simulink model "My_Model"  (R2022a)
settings: Solver=VariableStepAuto  StartTime=0.0  StopTime=10.0  RelTol=1e-3
libraries: neural x1294, spsSeriesRLCBranchLib x16, spsDiodeLib x14, spsMosfetLib x9, spsVoltageMeasurementLib x9, powerlib_extras x8, spsThreePhaseVIMeasurementLib x7, spsCurrentMeasurementLib x4, spsPVArrayLib x4, spsPWMGeneratorDCDCLib x4, spsTHDLib x4, spsThreePhaseParallelRLCBranchLib x3
(part 39 of 41)

== system My_Model/VSC Control/Current Regulator/7 layer network/Layer 5/IW{5,1} ==
  "pd{5,1}" : Inport  PortDimensions=2
      mask Display: e = 0.06;c1 = [120 230 180]/255;c2 = ([120 230 180]+0)/(256+128);c3 = ([120 230 180]+128)/(256+128);patch([0 1 1 0],[0 0 1 1],c1);patch([0 1 1 1-e 1-e 0+e],[0 0 1 1-e 0+e 0+e],c2);patch([0 0 1 1-e 0+e 0+e],[0 1 1 1-e 1-e 0+e],c3);plot([0 1 1 0 0],[0 0 1 1 0]);
  "IW{5,1}(1,:)'" : Constant  Value=[0.2265183678603188421885050729542854242026805877685546875;-0.080454707579343642809277525884681381285190582275390625]
      mask Display: e = 0.06;c1 = [120 150 230]/255;c2 = ([120 150 230]+0)/383;c3 = ([120 150 230]+128)/383;patch([0 1 1 0],[0 0 1 1],c1);patch([0 1 1 1-e 1-e 0+e],[0 0 1 1-e 0+e 0+e],c2);patch([0 0 1 1-e 0+e 0+e],[0 1 1 1-e 1-e 0+e],c3);plot([0 1 1 0 0],[0 0 1 1 0]);disp('Weights');
  "IW{5,1}(10,:)'" : Constant  Value=[-0.1422788353639719283183495690536801703274250030517578125;-0.07623245493874390710242749946701223962008953094482421875]
      mask Display: e = 0.06;c1 = [120 150 230]/255;c2 = ([120 150 230]+0)/383;c3 = ([120 150 230]+128)/383;patch([0 1 1 0],[0 0 1 1],c1);patch([0 1 1 1-e 1-e 0+e],[0 0 1 1-e 0+e 0+e],c2);patch([0 0 1 1-e 0+e 0+e],[0 1 1 1-e 1-e 0+e],c3);plot([0 1 1 0 0],[0 0 1 1 0]);disp('Weights');
  "IW{5,1}(2,:)'" : Constant  Value=[-0.4991813426266704656342199086793698370456695556640625;0.0282721598553938892328663001762834028340876102447509765625]
      mask Display: e = 0.06;c1 = [120 150 230]/255;c2 = ([120 150 230]+0)/383;c3 = ([120 150 230]+128)/383;patch([0 1 1 0],[0 0 1 1],c1);patch([0 1 1 1-e 1-e 0+e],[0 0 1 1-e 0+e 0+e],c2);patch([0 0 1 1-e 0+e 0+e],[0 1 1 1-e 1-e 0+e],c3);plot([0 1 1 0 0],[0 0 1 1 0]);disp('Weights');
  "IW{5,1}(3,:)'" : Constant  Value=[0.1044406469762407529966452557346201501786708831787109375;0.046202458042315097674901380742085166275501251220703125]
      mask Display: e = 0.06;c1 = [120 150 230]/255;c2 = ([120 150 230]+0)/383;c3 = ([120 150 230]+128)/383;patch([0 1 1 0],[0 0 1 1],c1);patch([0 1 1 1-e 1-e 0+e],[0 0 1 1-e 0+e 0+e],c2);patch([0 0 1 1-e 0+e 0+e],[0 1 1 1-e 1-e 0+e],c3);plot([0 1 1 0 0],[0 0 1 1 0]);disp('Weights');
  "IW{5,1}(4,:)'" : Constant  Value=[0.072802141329844138883942150641814805567264556884765625;-0.1804228821812341732044870923346024937927722930908203125]
      mask Display: e = 0.06;c1 = [120 150 230]/255;c2 = ([120 150 230]+0)/383;c3 = ([120 150 230]+128)/383;patch([0 1 1 0],[0 0 1 1],c1);patch([0 1 1 1-e 1-e 0+e],[0 0 1 1-e 0+e 0+e],c2);patch([0 0 1 1-e 0+e 0+e],[0 1 1 1-e 1-e 0+e],c3);plot([0 1 1 0 0],[0 0 1 1 0]);disp('Weights');
  "IW{5,1}(5,:)'" : Constant  Value=[-0.098564433750983615478702404288924299180507659912109375;-0.088427141857044144757082904106937348842620849609375]
      mask Display: e = 0.06;c1 = [120 150 230]/255;c2 = ([120 150 230]+0)/383;c3 = ([120 150 230]+128)/383;patch([0 1 1 0],[0 0 1 1],c1);patch([0 1 1 1-e 1-e 0+e],[0 0 1 1-e 0+e 0+e],c2);patch([0 0 1 1-e 0+e 0+e],[0 1 1 1-e 1-e 0+e],c3);plot([0 1 1 0 0],[0 0 1 1 0]);disp('Weights');
  "IW{5,1}(6,:)'" : Constant  Value=[-0.3674258864948158898044994202791713178157806396484375;0.0169846715856297354740878091661215876229107379913330078125]
      mask Display: e = 0.06;c1 = [120 150 230]/255;c2 = ([120 150 230]+0)/383;c3 = ([120 150 230]+128)/383;patch([0 1 1 0],[0 0 1 1],c1);patch([0 1 1 1-e 1-e 0+e],[0 0 1 1-e 0+e 0+e],c2);patch([0 0 1 1-e 0+e 0+e],[0 1 1 1-e 1-e 0+e],c3);plot([0 1 1 0 0],[0 0 1 1 0]);disp('Weights');
  "IW{5,1}(7,:)'" : Constant  Value=[0.4141842211099089343662171813775785267353057861328125;0.11901346031348351839351806802369537763297557830810546875]
      mask Display: e = 0.06;c1 = [120 150 230]/255;c2 = ([120 150 230]+0)/383;c3 = ([120 150 230]+128)/383;patch([0 1 1 0],[0 0 1 1],c1);patch([0 1 1 1-e 1-e 0+e],[0 0 1 1-e 0+e 0+e],c2);patch([0 0 1 1-e 0+e 0+e],[0 1 1 1-e 1-e 0+e],c3);plot([0 1 1 0 0],[0 0 1 1 0]);disp('Weights');
  "IW{5,1}(8,:)'" : Constant  Value=[-0.1725725080176267189902006293777958489954471588134765625;0.272154231131515211838944878763868473470211029052734375]
      mask Display: e = 0.06;c1 = [120 150 230]/255;c2 = ([120 150 230]+0)/383;c3 = ([120 150 230]+128)/383;patch([0 1 1 0],[0 0 1 1],c1);patch([0 1 1 1-e 1-e 0+e],[0 0 1 1-e 0+e 0+e],c2);patch([0 0 1 1-e 0+e 0+e],[0 1 1 1-e 1-e 0+e],c3);plot([0 1 1 0 0],[0 0 1 1 0]);disp('Weights');
  "IW{5,1}(9,:)'" : Constant  Value=[-0.2126507656600488405107540756944217719137668609619140625;0.11513492898073794667990199513951665721833705902099609375]
      mask Display: e = 0.06;c1 = [120 150 230]/255;c2 = ([120 150 230]+0)/383;c3 = ([120 150 230]+128)/383;patch([0 1 1 0],[0 0 1 1],c1);patch([0 1 1 1-e 1-e 0+e],[0 0 1 1-e 0+e 0+e],c2);patch([0 0 1 1-e 0+e 0+e],[0 1 1 1-e 1-e 0+e],c3);plot([0 1 1 0 0],[0 0 1 1 0]);disp('Weights');
  Mux : Mux  Inputs=10
      mask Display: e = 0.06;c1 = [120 150 230]/255;c2 = ([120 150 230]+0)/383;c3 = ([120 150 230]+128)/383;patch([0 1 1 0],[0 0 1 1],c1);patch([0 1 1 1-e 1-e 0+e],[0 0 1 1-e 0+e 0+e],c2);patch([0 0 1 1-e 0+e 0+e],[0 1 1 1-e 1-e 0+e],c3);plot([0 1 1 0 0],[0 0 1 1 0]);disp('Mux');
  dotprod{1..10} (10 alike) : neural/Weight Functions/dotprod
  "iz{5,1}" : Outport
      mask Display: e = 0.06;c1 = [120 230 180]/255;c2 = ([120 230 180]+0)/(256+128);c3 = ([120 230 180]+128)/(256+128);patch([0 1 1 0],[0 0 1 1],c1);patch([0 1 1 1-e 1-e 0+e],[0 0 1 1-e 0+e 0+e],c2);patch([0 0 1 1-e 0+e 0+e],[0 1 1 1-e 1-e 0+e],c3);plot([0 1 1 0 0],[0 0 1 1 0]);
  wires:
  "IW{5,1}(1,:)'"/1 -> dotprod1/1
  "pd{5,1}"/1 -> dotprod1/2, dotprod2/2, dotprod3/2, dotprod4/2, dotprod5/2, dotprod6/2, dotprod7/2, dotprod8/2, dotprod9/2, dotprod10/2
  dotprod1/1 -> Mux/1
  "IW{5,1}(2,:)'"/1 -> dotprod2/1
  dotprod2/1 -> Mux/2
  "IW{5,1}(3,:)'"/1 -> dotprod3/1
  dotprod3/1 -> Mux/3
  "IW{5,1}(4,:)'"/1 -> dotprod4/1
  dotprod4/1 -> Mux/4
  "IW{5,1}(5,:)'"/1 -> dotprod5/1
  dotprod5/1 -> Mux/5
  "IW{5,1}(6,:)'"/1 -> dotprod6/1
  dotprod6/1 -> Mux/6
  "IW{5,1}(7,:)'"/1 -> dotprod7/1
  dotprod7/1 -> Mux/7
  "IW{5,1}(8,:)'"/1 -> dotprod8/1
  dotprod8/1 -> Mux/8
  "IW{5,1}(9,:)'"/1 -> dotprod9/1
  dotprod9/1 -> Mux/9
  "IW{5,1}(10,:)'"/1 -> dotprod10/1
  dotprod10/1 -> Mux/10
  Mux/1 -> "iz{5,1}"/1

== system My_Model/VSC Control/Current Regulator/7 layer network/Layer 5/LW{5,1} ==
  "ad{5,1}" : Inport  PortDimensions=5
      mask Display: e = 0.06;c1 = [120 230 180]/255;c2 = ([120 230 180]+0)/(256+128);c3 = ([120 230 180]+128)/(256+128);patch([0 1 1 0],[0 0 1 1],c1);patch([0 1 1 1-e 1-e 0+e],[0 0 1 1-e 0+e 0+e],c2);patch([0 0 1 1-e 0+e 0+e],[0 1 1 1-e 1-e 0+e],c3);plot([0 1 1 0 0],[0 0 1 1 0]);
  "IW{5,1}(1,:)'" : Constant  Value=[0.9171581622873168360143836252973414957523345947265625;-0.97707391492595940807319720988743938505649566650390625;-0.0210179710971976907440961213069385848939418792724609375;1.1725033658274852665925891415099613368511199951171875;-0.130605738254601033698776291203103028237819671630859375]
      mask Display: e = 0.06;c1 = [120 150 230]/255;c2 = ([120 150 230]+0)/383;c3 = ([120 150 230]+128)/383;patch([0 1 1 0],[0 0 1 1],c1);patch([0 1 1 1-e 1-e 0+e],[0 0 1 1-e 0+e 0+e],c2);patch([0 0 1 1-e 0+e 0+e],[0 1 1 1-e 1-e 0+e],c3);plot([0 1 1 0 0],[0 0 1 1 0]);disp('weights');
  "IW{5,1}(10,:)'" : Constant  Value=[-0.99600515073955653289061729083186946809291839599609375;-0.167577225793884732052418939929339103400707244873046875;0.95217978635098254880375634456868283450603485107421875;-0.7188933838155431299554720681044273078441619873046875;-0.831292356468587900764077858184464275836944580078125]
      mask Display: e = 0.06;c1 = [120 150 230]/255;c2 = ([120 150 230]+0)/383;c3 = ([120 150 230]+128)/383;patch([0 1 1 0],[0 0 1 1],c1);patch([0 1 1 1-e 1-e 0+e],[0 0 1 1-e 0+e 0+e],c2);patch([0 0 1 1-e 0+e 0+e],[0 1 1 1-e 1-e 0+e],c3);plot([0 1 1 0 0],[0 0 1 1 0]);disp('weights');
  "IW{5,1}(2,:)'" : Constant  Value=[-0.99814062980683948556048790123895741999149322509765625;0.354655699276410107945167737852898426353931427001953125;-1.1738397879619137942341922098421491682529449462890625;-0.8104641536272778612470801817835308611392974853515625;-0.18663113226859640025878661617753095924854278564453125]
      mask Display: e = 0.06;c1 = [120 150 230]/255;c2 = ([120 150 230]+0)/383;c3 = ([120 150 230]+128)/383;patch([0 1 1 0],[0 0 1 1],c1);patch([0 1 1 1-e 1-e 0+e],[0 0 1 1-e 0+e 0+e],c2);patch([0 0 1 1-e 0+e 0+e],[0 1 1 1-e 1-e 0+e],c3);plot([0 1 1 0 0],[0 0 1 1 0]);disp('weights');
  "IW{5,1}(3,:)'" : Constant  Value=[-1.0672547131758600702511330382549203932285308837890625;0.82489928776503373963890908271423541009426116943359375;0.97161303536051224494229927586275152862071990966796875;-0.578809431848783528806734466343186795711517333984375;1.1398055234981889771717078474466688930988311767578125]
      mask Display: e = 0.06;c1 = [120 150 230]/255;c2 = ([120 150 230]+0)/383;c3 = ([120 150 230]+128)/383;patch([0 1 1 0],[0 0 1 1],c1);patch([0 1 1 1-e 1-e 0+e],[0 0 1 1-e 0+e 0+e],c2);patch([0 0 1 1-e 0+e 0+e],[0 1 1 1-e 1-e 0+e],c3);plot([0 1 1 0 0],[0 0 1 1 0]);disp('weights');
  "IW{5,1}(4,:)'" : Constant  Value=[-0.94982133378153721370296125314780510962009429931640625;1.1679083219168562290946056236862204968929290771484375;-1.057736150922272688745806590304709970951080322265625;0.98685120281576044209970177689683623611927032470703125;0.303639924542568107046491832079482264816761016845703125]
      mask Display: e = 0.06;c1 = [120 150 230]/255;c2 = ([120 150 230]+0)/383;c3 = ([120 150 230]+128)/383;patch([0 1 1 0],[0 0 1 1],c1);patch([0 1 1 1-e 1-e 0+e],[0 0 1 1-e 0+e 0+e],c2);patch([0 0 1 1-e 0+e 0+e],[0 1 1 1-e 1-e 0+e],c3);plot([0 1 1 0 0],[0 0 1 1 0]);disp('weights');
  "IW{5,1}(5,:)'" : Constant  Value=[-1.0417328454976433338430297226295806467533111572265625;0.2087784483975625715590496156437438912689685821533203125;-0.1995658207885550872173752168237115256488323211669921875;0.28455370307110638972147853564820252358913421630859375;0.5979985260828233339935877665993757545948028564453125]
      mask Display: e = 0.06;c1 = [120 150 230]/255;c2 = ([120 150 230]+0)/383;c3 = ([120 150 230]+128)/383;patch([0 1 1 0],[0 0 1 1],c1);patch([0 1 1 1-e 1-e 0+e],[0 0 1 1-e 0+e 0+e],c2);patch([0 0 1 1-e 0+e 0+e],[0 1 1 1-e 1-e 0+e],c3);plot([0 1 1 0 0],[0 0 1 1 0]);disp('weights');
  "IW{5,1}(6,:)'" : Constant  Value=[-0.411010294145512100616457473734044469892978668212890625;1.197115103363101784594846321851946413516998291015625;0.79345318280653354126030762927257455885410308837890625;0.009881410922908513694284948769563925452530384063720703125;0.53039145325024306121264316971064545214176177978515625]
      mask Display: e = 0.06;c1 = [120 150 230]/255;c2 = ([120 150 230]+0)/383;c3 = ([120 150 230]+128)/383;patch([0 1 1 0],[0 0 1 1],c1);patch([0 1 1 1-e 1-e 0+e],[0 0 1 1-e 0+e 0+e],c2);patch([0 0 1 1-e 0+e 0+e],[0 1 1 1-e 1-e 0+e],c3);plot([0 1 1 0 0],[0 0 1 1 0]);disp('weights');
  "IW{5,1}(7,:)'" : Constant  Value=[-0.6802913607797160810974901323788799345493316650390625;0.2076033210000148010454523728185449726879596710205078125;-0.35479842057045851699825789182796142995357513427734375;0.35408602528381505347709889974794350564479827880859375;-0.490501379559078076741940321880974806845188140869140625]
      mask Display: e = 0.06;c1 = [120 150 230]/255;c2 = ([120 150 230]+0)/383;c3 = ([120 150 230]+128)/383;patch([0 1 1 0],[0 0 1 1],c1);patch([0 1 1 1-e 1-e 0+e],[0 0 1 1-e 0+e 0+e],c2);patch([0 0 1 1-e 0+e 0+e],[0 1 1 1-e 1-e 0+e],c3);plot([0 1 1 0 0],[0 0 1 1 0]);disp('weights');
  "IW{5,1}(8,:)'" : Constant  Value=[-1.1781079921274797417396484888740815222263336181640625;0.03729631809679491427633735156632610596716403961181640625;0.27379991360773237030201698871678672730922698974609375;0.77074107115669654444189973219181410968303680419921875;0.041084841969233919234394392105969018302857875823974609375]
      mask Display: e = 0.06;c1 = [120 150 230]/255;c2 = ([120 150 230]+0)/383;c3 = ([120 150 230]+128)/383;patch([0 1 1 0],[0 0 1 1],c1);patch([0 1 1 1-e 1-e 0+e],[0 0 1 1-e 0+e 0+e],c2);patch([0 0 1 1-e 0+e 0+e],[0 1 1 1-e 1-e 0+e],c3);plot([0 1 1 0 0],[0 0 1 1 0]);disp('weights');
  "IW{5,1}(9,:)'" : Constant  Value=[0.07845840624283091646606891345072654075920581817626953125;-0.422066310984252568427876894929795525968074798583984375;0.7903163990136097272198867358383722603321075439453125;0.1485772442357067013585236736616934649646282196044921875;0.1708029115967119315744326968342647887766361236572265625]
      mask Display: e = 0.06;c1 = [120 150 230]/255;c2 = ([120 150 230]+0)/383;c3 = ([120 150 230]+128)/383;patch([0 1 1 0],[0 0 1 1],c1);patch([0 1 1 1-e 1-e 0+e],[0 0 1 1-e 0+e 0+e],c2);patch([0 0 1 1-e 0+e 0+e],[0 1 1 1-e 1-e 0+e],c3);plot([0 1 1 0 0],[0 0 1 1 0]);disp('weights');
  Mux : Mux  Inputs=10
      mask Display: e = 0.06;c1 = [120 150 230]/255;c2 = ([120 150 230]+0)/383;c3 = ([120 150 230]+128)/383;patch([0 1 1 0],[0 0 1 1],c1);patch([0 1 1 1-e 1-e 0+e],[0 0 1 1-e 0+e 0+e],c2);patch([0 0 1 1-e 0+e 0+e],[0 1 1 1-e 1-e 0+e],c3);plot([0 1 1 0 0],[0 0 1 1 0]);disp('Mux');
  dotprod{1..10} (10 alike) : neural/Weight Functions/dotprod
  "lz{5,1}" : Outport
      mask Display: e = 0.06;c1 = [120 230 180]/255;c2 = ([120 230 180]+0)/(256+128);c3 = ([120 230 180]+128)/(256+128);patch([0 1 1 0],[0 0 1 1],c1);patch([0 1 1 1-e 1-e 0+e],[0 0 1 1-e 0+e 0+e],c2);patch([0 0 1 1-e 0+e 0+e],[0 1 1 1-e 1-e 0+e],c3);plot([0 1 1 0 0],[0 0 1 1 0]);
  wires:
  "IW{5,1}(1,:)'"/1 -> dotprod1/1
  "ad{5,1}"/1 -> dotprod1/2, dotprod2/2, dotprod3/2, dotprod4/2, dotprod5/2, dotprod6/2, dotprod7/2, dotprod8/2, dotprod9/2, dotprod10/2
  dotprod1/1 -> Mux/1
  "IW{5,1}(2,:)'"/1 -> dotprod2/1
  dotprod2/1 -> Mux/2
  "IW{5,1}(3,:)'"/1 -> dotprod3/1
  dotprod3/1 -> Mux/3
  "IW{5,1}(4,:)'"/1 -> dotprod4/1
  dotprod4/1 -> Mux/4
  "IW{5,1}(5,:)'"/1 -> dotprod5/1
  dotprod5/1 -> Mux/5
  "IW{5,1}(6,:)'"/1 -> dotprod6/1
  dotprod6/1 -> Mux/6
  "IW{5,1}(7,:)'"/1 -> dotprod7/1
  dotprod7/1 -> Mux/7
  "IW{5,1}(8,:)'"/1 -> dotprod8/1
  dotprod8/1 -> Mux/8
  "IW{5,1}(9,:)'"/1 -> dotprod9/1
  dotprod9/1 -> Mux/9
  "IW{5,1}(10,:)'"/1 -> dotprod10/1
  dotprod10/1 -> Mux/10
  Mux/1 -> "lz{5,1}"/1

== system My_Model/VSC Control/Current Regulator/7 layer network/Layer 5/LW{5,2} ==
  "ad{5,2}" : Inport  PortDimensions=10
      mask Display: e = 0.06;c1 = [120 230 180]/255;c2 = ([120 230 180]+0)/(256+128);c3 = ([120 230 180]+128)/(256+128);patch([0 1 1 0],[0 0 1 1],c1);patch([0 1 1 1-e 1-e 0+e],[0 0 1 1-e 0+e 0+e],c2);patch([0 0 1 1-e 0+e 0+e],[0 1 1 1-e 1-e 0+e],c3);plot([0 1 1 0 0],[0 0 1 1 0]);
  "IW{5,2}(1,:)'" : Constant  Value=[0.1684578037809467410124142361382837407290935516357421875;-0.193004051966780443283511203844682313501834869384765625;-0.7569737646740828385105714914971031248569488525390625;0.46291825933074892684970791378873400390148162841796875;1.000716263096052660586110505391843616962432861328125;1.14373966364727674971391024882905185222625732421875;0.048892907784722404451738242414648993872106075286865234375;0.14834399129137321171612029502284713089466094970703125;-0.265260424955228557575281911340425722301006317138671875;-0.56311916317580223978467302003991790115833282470703125]
      mask Display: e = 0.06;c1 = [120 150 230]/255;c2 = ([120 150 230]+0)/383;c3 = ([120 150 230]+128)/383;patch([0 1 1 0],[0 0 1 1],c1);patch([0 1 1 1-e 1-e 0+e],[0 0 1 1-e 0+e 0+e],c2);patch([0 0 1 1-e 0+e 0+e],[0 1 1 1-e 1-e 0+e],c3);plot([0 1 1 0 0],[0 0 1 1 0]);disp('weights');
  "IW{5,2}(10,:)'" : Constant  Value=[0.5965895726190824088774888878106139600276947021484375;-1.109654058320999059361611216445453464984893798828125;-0.92939814722662983381695767093333415687084197998046875;0.06581594925990268130089333453724975697696208953857421875;0.87560511493496473445219407949480228126049041748046875;0.402556470821988809927205466010491363704204559326171875;0.08116409296593292410637587863675435073673725128173828125;-0.476045626559129242405532522752764634788036346435546875;-0.59508999328593137345677632765728048980236053466796875;-1.208177901676958043708509649150073528289794921875]
      mask Display: e = 0.06;c1 = [120 150 230]/255;c2 = ([120 150 230]+0)/383;c3 = ([120 150 230]+128)/383;patch([0 1 1 0],[0 0 1 1],c1);patch([0 1 1 1-e 1-e 0+e],[0 0 1 1-e 0+e 0+e],c2);patch([0 0 1 1-e 0+e 0+e],[0 1 1 1-e 1-e 0+e],c3);plot([0 1 1 0 0],[0 0 1 1 0]);disp('weights');
  "IW{5,2}(2,:)'" : Constant  Value=[0.5392099312023106438829245234956033527851104736328125;0.5284626071393976332046804600395262241363525390625;0.9226219027712969644738905117264948785305023193359375;0.295586522777884663781833296525292098522186279296875;-1.0818364442210697262680696439929306507110595703125;1.3388256505409283914076468136045150458812713623046875;-0.90283403273780560294170527413371019065380096435546875;0.492871626511317051377858433625078760087490081787109375;0.89484365751269134836576313318801112473011016845703125;-0.1939595109481083989866334604812436737120151519775390625]
      mask Display: e = 0.06;c1 = [120 150 230]/255;c2 = ([120 150 230]+0)/383;c3 = ([120 150 230]+128)/383;patch([0 1 1 0],[0 0 1 1],c1);patch([0 1 1 1-e 1-e 0+e],[0 0 1 1-e 0+e 0+e],c2);patch([0 0 1 1-e 0+e 0+e],[0 1 1 1-e 1-e 0+e],c3);plot([0 1 1 0 0],[0 0 1 1 0]);disp('weights');
  "IW{5,2}(3,:)'" : Constant  Value=[-0.1726404059552293090984420587119529955089092254638671875;1.0776924203056370554776322023826651275157928466796875;-1.1937432381249148960478123626671731472015380859375;-1.0727438918897720387946037590154446661472320556640625;0.9981173788149868553176702334894798696041107177734375;0.0277089161893979696316137051326222717761993408203125;1.065316039319306629096217875485308468341827392578125;-0.357304648277443515080875613421085290610790252685546875;-0.26755186309950940160007348822546191513538360595703125;-0.91913923080617421224047802752465941011905670166015625]
      mask Display: e = 0.06;c1 = [120 150 230]/255;c2 = ([120 150 230]+0)/383;c3 = ([120 150 230]+128)/383;patch([0 1 1 0],[0 0 1 1],c1);patch([0 1 1 1-e 1-e 0+e],[0 0 1 1-e 0+e 0+e],c2);patch([0 0 1 1-e 0+e 0+e],[0 1 1 1-e 1-e 0+e],c3);plot([0 1 1 0 0],[0 0 1 1 0]);disp('weights');
  "IW{5,2}(4,:)'" : Constant  Value=[0.816010046257328536256636652979068458080291748046875;0.68459856295321219743499341348069719970226287841796875;0.89589179574365884750619670739979483187198638916015625;-1.02853605870084141571396685321815311908721923828125;-0.8918674167578901634811927578994072973728179931640625;-0.53748834516843480013648104431922547519207000732421875;0.209761195044842085888348037769901566207408905029296875;-0.5887706365142033604342941544018685817718505859375;-0.222808741470218285574134142734692431986331939697265625;0.00754126643356810809348811375230070552788674831390380859375]
      mask Display: e = 0.06;c1 = [120 150 230]/255;c2 = ([120 150 230]+0)/383;c3 = ([120 150 230]+128)/383;patch([0 1 1 0],[0 0 1 1],c1);patch([0 1 1 1-e 1-e 0+e],[0 0 1 1-e 0+e 0+e],c2);patch([0 0 1 1-e 0+e 0+e],[0 1 1 1-e 1-e 0+e],c3);plot([0 1 1 0 0],[0 0 1 1 0]);disp('weights');
  "IW{5,2}(5,:)'" : Constant  Value=[0.708507577507914820813539336086250841617584228515625;0.6318384603124085341363525003544054925441741943359375;-1.3059952879512539691830852461862377822399139404296875;-1.066632472389412722435508840135298669338226318359375;0.049698052881103682576480196075863204896450042724609375;-1.229398698707528492235496742068789899349212646484375;-0.1822713071628439263083265586828929372131824493408203125;0.241133002219878156413557235282496549189090728759765625;-0.443578298026761130845585512361139990389347076416015625;0.6318249462983802633431196227320469915866851806640625]
      mask Display: e = 0.06;c1 = [120 150 230]/255;c2 = ([120 150 230]+0)/383;c3 = ([120 150 230]+128)/383;patch([0 1 1 0],[0 0 1 1],c1);patch([0 1 1 1-e 1-e 0+e],[0 0 1 1-e 0+e 0+e],c2);patch([0 0 1 1-e 0+e 0+e],[0 1 1 1-e 1-e 0+e],c3);plot([0 1 1 0 0],[0 0 1 1 0]);disp('weights');
  "IW{5,2}(6,:)'" : Constant  Value=[-0.341533336982904611733857791477930732071399688720703125;-0.94716798187301531886106431556981988251209259033203125;0.40817790070221582343634736389503814280033111572265625;-1.1645967613063785695004526132834143936634063720703125;-0.863973627364388097049641146440990269184112548828125;0.0240787013609295823257649971083083073608577251434326171875;1.064216682141272851680469102575443685054779052734375;0.87811788686155722860604555535246618092060089111328125;-0.8632119916674978465920275993994437158107757568359375;-0.621833169879618008479837953927926719188690185546875]
      mask Display: e = 0.06;c1 = [120 150 230]/255;c2 = ([120 150 230]+0)/383;c3 = ([120 150 230]+128)/383;patch([0 1 1 0],[0 0 1 1],c1);patch([0 1 1 1-e 1-e 0+e],[0 0 1 1-e 0+e 0+e],c2);patch([0 0 1 1-e 0+e 0+e],[0 1 1 1-e 1-e 0+e],c3);plot([0 1 1 0 0],[0 0 1 1 0]);disp('weights');
  "IW{5,2}(7,:)'" : Constant  Value=[-0.14729418465331567400511403320706449449062347412109375;-0.34746659552439862483907973000896163284778594970703125;0.005906531899335795525451953125184445525519549846649169921875;-0.198031562781192160827004045131616294384002685546875;0.1845816164199503839338234456590726040303707122802734375;0.2493414791277918929335299935701186768710613250732421875;0.496537373225766354156718307422124780714511871337890625;-0.273671814571639526736390735095483250916004180908203125;-0.77881973615030830604410994055797345936298370361328125;0.90546099911025390571950310913962312042713165283203125]
      mask Display: e = 0.06;c1 = [120 150 230]/255;c2 = ([120 150 230]+0)/383;c3 = ([120 150 230]+128)/383;patch([0 1 1 0],[0 0 1 1],c1);patch([0 1 1 1-e 1-e 0+e],[0 0 1 1-e 0+e 0+e],c2);patch([0 0 1 1-e 0+e 0+e],[0 1 1 1-e 1-e 0+e],c3);plot([0 1 1 0 0],[0 0 1 1 0]);disp('weights');
  "IW{5,2}(8,:)'" : Constant  Value=[-0.273999752744912006274802251937217079102993011474609375;0.2193199636475850200501014342080452479422092437744140625;-0.68027994906388833395993742669816128909587860107421875;0.80160613802942837224918548599816858768463134765625;-1.1951697068245341615266852386412210762500762939453125;0.63427707178833403478535046815522946417331695556640625;-0.1159513192323429198182793697924353182315826416015625;-0.93455582119741809066226778668351471424102783203125;-0.99679512560920613406523216326604597270488739013671875;-1.027446353007799739742722522350959479808807373046875]
      mask Display: e = 0.06;c1 = [120 150 230]/255;c2 = ([120 150 230]+0)/383;c3 = ([120 150 230]+128)/383;patch([0 1 1 0],[0 0 1 1],c1);patch([0 1 1 1-e 1-e 0+e],[0 0 1 1-e 0+e 0+e],c2);patch([0 0 1 1-e 0+e 0+e],[0 1 1 1-e 1-e 0+e],c3);plot([0 1 1 0 0],[0 0 1 1 0]);disp('weights');
  "IW{5,2}(9,:)'" : Constant  Value=[0.72121309021742663336596024237223900854587554931640625;-0.1016887643432220211803240772496792487800121307373046875;0.2126081411526652420462824011337943375110626220703125;0.350058599740678266787341499366448260843753814697265625;0.688746733470050553904684420558623969554901123046875;-1.0332141310706652870265997989918105304241180419921875;0.85423428410211921235628551585250534117221832275390625;-0.1139430891934676559618111468807910569012165069580078125;-0.2125492359396747021893503415412851609289646148681640625;-0.2419182777835253983500507501958054490387439727783203125]
      mask Display: e = 0.06;c1 = [120 150 230]/255;c2 = ([120 150 230]+0)/383;c3 = ([120 150 230]+128)/383;patch([0 1 1 0],[0 0 1 1],c1);patch([0 1 1 1-e 1-e 0+e],[0 0 1 1-e 0+e 0+e],c2);patch([0 0 1 1-e 0+e 0+e],[0 1 1 1-e 1-e 0+e],c3);plot([0 1 1 0 0],[0 0 1 1 0]);disp('weights');
  Mux : Mux  Inputs=10
      mask Display: e = 0.06;c1 = [120 150 230]/255;c2 = ([120 150 230]+0)/383;c3 = ([120 150 230]+128)/383;patch([0 1 1 0],[0 0 1 1],c1);patch([0 1 1 1-e 1-e 0+e],[0 0 1 1-e 0+e 0+e],c2);patch([0 0 1 1-e 0+e 0+e],[0 1 1 1-e 1-e 0+e],c3);plot([0 1 1 0 0],[0 0 1 1 0]);disp('Mux');
  dotprod{1..10} (10 alike) : neural/Weight Functions/dotprod
  "lz{5,2}" : Outport
      mask Display: e = 0.06;c1 = [120 230 180]/255;c2 = ([120 230 180]+0)/(256+128);c3 = ([120 230 180]+128)/(256+128);patch([0 1 1 0],[0 0 1 1],c1);patch([0 1 1 1-e 1-e 0+e],[0 0 1 1-e 0+e 0+e],c2);patch([0 0 1 1-e 0+e 0+e],[0 1 1 1-e 1-e 0+e],c3);plot([0 1 1 0 0],[0 0 1 1 0]);
  wires:
  "IW{5,2}(1,:)'"/1 -> dotprod1/1
  "ad{5,2}"/1 -> dotprod1/2, dotprod2/2, dotprod3/2, dotprod4/2, dotprod5/2, dotprod6/2, dotprod7/2, dotprod8/2, dotprod9/2, dotprod10/2
  dotprod1/1 -> Mux/1
  "IW{5,2}(2,:)'"/1 -> dotprod2/1
  dotprod2/1 -> Mux/2
  "IW{5,2}(3,:)'"/1 -> dotprod3/1
  dotprod3/1 -> Mux/3
  "IW{5,2}(4,:)'"/1 -> dotprod4/1
  dotprod4/1 -> Mux/4
  "IW{5,2}(5,:)'"/1 -> dotprod5/1
  dotprod5/1 -> Mux/5
  "IW{5,2}(6,:)'"/1 -> dotprod6/1
  dotprod6/1 -> Mux/6
  "IW{5,2}(7,:)'"/1 -> dotprod7/1
  dotprod7/1 -> Mux/7
  "IW{5,2}(8,:)'"/1 -> dotprod8/1
  dotprod8/1 -> Mux/8
  "IW{5,2}(9,:)'"/1 -> dotprod9/1
  dotprod9/1 -> Mux/9
  "IW{5,2}(10,:)'"/1 -> dotprod10/1
  dotprod10/1 -> Mux/10
  Mux/1 -> "lz{5,2}"/1

== system My_Model/VSC Control/Current Regulator/7 layer network/Layer 5/LW{5,3} ==
  "ad{5,3}" : Inport  PortDimensions=20
      mask Display: e = 0.06;c1 = [120 230 180]/255;c2 = ([120 230 180]+0)/(256+128);c3 = ([120 230 180]+128)/(256+128);patch([0 1 1 0],[0 0 1 1],c1);patch([0 1 1 1-e 1-e 0+e],[0 0 1 1-e 0+e 0+e],c2);patch([0 0 1 1-e 0+e 0+e],[0 1 1 1-e 1-e 0+e],c3);plot([0 1 1 0 0],[0 0 1 1 0]);
  "IW{5,3}(1,:)'" : Constant  Value=[-0.7739352357042348362625716617912985384464263916015625;-0.77039040031364691696325053271721117198467254638671875;-0.194426366768218616964958300741272978484630584716796875;-0.7514822618890584227102635850314982235431671142578125;-0.464584934444699892974739441342535428702831268310546875;-0.490136343053946765824235853870050050318241119384765625;1.2010206804188394702492814758443273603916168212890625;0.114183614101492414416583187630749307572841644287109375;0.00930962456358271940592974402761683450080454349517822265625;0.08925580014502322578895388005548738874495029449462890625;-0.1314709305617100809637776137606124393641948699951171875;1.328545970208529158895771615789271891117095947265625;-0.9633599949989513078207892249338328838348388671875;-0.741896333933734997145847955835051834583282470703125;0.01311264882287951037687090405370327061973512172698974609375;0.99315051108612995012236979164299555122852325439453125;-0.50339308809133986866157783879316411912441253662109375;-0.133186954343675389988987944889231584966182708740234375;0.96790429482423279150538064641295932233333587646484375;-0.5977605605644082942262684809975326061248779296875]
      mask Display: e = 0.06;c1 = [120 150 230]/255;c2 = ([120 150 230]+0)/383;c3 = ([120 150 230]+128)/383;patch([0 1 1 0],[0 0 1 1],c1);patch([0 1 1 1-e 1-e 0+e],[0 0 1 1-e 0+e 0+e],c2);patch([0 0 1 1-e 0+e 0+e],[0 1 1 1-e 1-e 0+e],c3);plot([0 1 1 0 0],[0 0 1 1 0]);disp('weights');
  "IW{5,3}(10,:)'" : Constant  Value=[1.100068863723112411179272385197691619396209716796875;1.12184633477385187205754846218042075634002685546875;0.68232110416673197317294352615135721862316131591796875;0.226277370415800038738751709388452582061290740966796875;-0.756044104448321707678815073450095951557159423828125;1.1433894393910823961135747595108114182949066162109375;0.32006905710428579237003532398375682532787322998046875;-0.92750324975228715107533616901491768658161163330078125;-1.1931697368768154898788225182215683162212371826171875;-1.093606973868940901439827939611859619617462158203125;-1.078509294300400878086065858951769769191741943359375;-0.5570902920817271120057512234780006110668182373046875;0.73218433092913970394732814384042285382747650146484375;0.8714188310587978048005197706515900790691375732421875;-0.58747394138984787570478829366038553416728973388671875;-1.0112522188888768415182539683883078396320343017578125;-0.436823632572289011211097431441885419189929962158203125;-0.5153288784599296956656644397298805415630340576171875;0.20909303197323503287208268375252373516559600830078125;-0.9004116887877222641378693879232741892337799072265625]
      mask Display: e = 0.06;c1 = [120 150 230]/255;c2 = ([120 150 230]+0)/383;c3 = ([120 150 230]+128)/383;patch([0 1 1 0],[0 0 1 1],c1);patch([0 1 1 1-e 1-e 0+e],[0 0 1 1-e 0+e 0+e],c2);patch([0 0 1 1-e 0+e 0+e],[0 1 1 1-e 1-e 0+e],c3);plot([0 1 1 0 0],[0 0 1 1 0]);disp('weights');
  "IW{5,3}(2,:)'" : Constant  Value=[-1.352248269026136373582858141162432730197906494140625;-0.04709242640835216431316467833312344737350940704345703125;1.2629285503316280969698937042267061769962310791015625;-0.3518417574942265257931239830213598906993865966796875;0.9733146926118647623837887294939719140529632568359375;-0.259809939053406602216256260362570174038410186767578125;0.87761338667890154141559833078645169734954833984375;-0.1587970503917780773495138646467239595949649810791015625;-0.4034010739377003051941983358119614422321319580078125;-0.60079121214464803468757736482075415551662445068359375;0.2179220368545104202784301605788641609251499176025390625;-0.59306053646582068683557054100674577057361602783203125;-0.273713299729888059896865115661057643592357635498046875;-0.12245090289223155288755862102334504015743732452392578125;-0.59124259218041108621122248223400674760341644287109375;1.1164366300777128770960189285688102245330810546875;0.053539562182813242585677215856776456348598003387451171875;0.68996497894668562533837530281743966042995452880859375;1.121524164967360182032507509575225412845611572265625;0.90219337805957244835752817380125634372234344482421875]
      mask Display: e = 0.06;c1 = [120 150 230]/255;c2 = ([120 150 230]+0)/383;c3 = ([120 150 230]+128)/383;patch([0 1 1 0],[0 0 1 1],c1);patch([0 1 1 1-e 1-e 0+e],[0 0 1 1-e 0+e 0+e],c2);patch([0 0 1 1-e 0+e 0+e],[0 1 1 1-e 1-e 0+e],c3);plot([0 1 1 0 0],[0 0 1 1 0]);disp('weights');
  "IW{5,3}(3,:)'" : Constant  Value=[-0.72830384921749791171663446220918558537960052490234375;-0.304004195509223140714283317720401100814342498779296875;0.60456151685986869726008308134623803198337554931640625;0.9472194065698669174224733069422654807567596435546875;-0.154112902304948118370475640404038131237030029296875;0.1266126948120616102499980115680955350399017333984375;0.573798902168273894375261079403571784496307373046875;-0.510049799637522394135658032610081136226654052734375;-0.94707479936752625437890173998312093317508697509765625;1.080633332147471481476941335131414234638214111328125;0.448709310694966501120717339290422387421131134033203125;0.229772802454730140642169544662465341389179229736328125;-0.2994881759333247739363059736206196248531341552734375;0.155479459410720444179077048829640261828899383544921875;0.600827651696863807018189618247561156749725341796875;0.488462649485105426805375827825628221035003662109375;-1.064578316952914605053592822514474391937255859375;-0.94162725485494025434718423639424145221710205078125;0.33783881308332175397168839481309987604618072509765625;-0.73026065707753529121504243448725901544094085693359375]
      mask Display: e = 0.06;c1 = [120 150 230]/255;c2 = ([120 150 230]+0)/383;c3 = ([120 150 230]+128)/383;patch([0 1 1 0],[0 0 1 1],c1);patch([0 1 1 1-e 1-e 0+e],[0 0 1 1-e 0+e 0+e],c2);patch([0 0 1 1-e 0+e 0+e],[0 1 1 1-e 1-e 0+e],c3);plot([0 1 1 0 0],[0 0 1 1 0]);disp('weights');
  "IW{5,3}(4,:)'" : Constant  Value=[-0.86629710940807636010418946170830167829990386962890625;0.0633018036493875058123848020841251127421855926513671875;-1.1484493500080439343236093918676488101482391357421875;0.84731985728977365912584218676784075796604156494140625;1.0099621485995646796851588078425265848636627197265625;-1.0488462000313212296731535388971678912639617919921875;-0.76829319223707415176249924115836620330810546875;0.002567804597515220381420686379669859888963401317596435546875;-0.8614838078794828657436255525681190192699432373046875;0.966433385068039996212974074296653270721435546875;0.5369096432910860361431559795164503157138824462890625;1.097379686591054781530374384601600468158721923828125;-0.85907236105435724748957682095351628959178924560546875;-1.0082796600259913422092949986108578741550445556640625;-0.59643031744419616746455403699656017124652862548828125;0.52590426328545325507235475015477277338504791259765625;0.57261239884450676473903740770765580236911773681640625;-0.93069087160195385077798846396035514771938323974609375;-0.5821858886357205165040795691311359405517578125;-0.146633552827470037271950786816887557506561279296875]
      mask Display: e = 0.06;c1 = [120 150 230]/255;c2 = ([120 150 230]+0)/383;c3 = ([120 150 230]+128)/383;patch([0 1 1 0],[0 0 1 1],c1);patch([0 1 1 1-e 1-e 0+e],[0 0 1 1-e 0+e 0+e],c2);patch([0 0 1 1-e 0+e 0+e],[0 1 1 1-e 1-e 0+e],c3);plot([0 1 1 0 0],[0 0 1 1 0]);disp('weights');
  "IW{5,3}(5,:)'" : Constant  Value=[-0.7049181519460760991790948537527583539485931396484375;-0.726205002243004660300584873766638338565826416015625;0.5525633598062851259413719162694178521633148193359375;-0.300026430743073058149406051597907207906246185302734375;-1.4347347712886271420273942567291669547557830810546875;0.1572840993115438568139552444336004555225372314453125;-0.425957616003774630630829278743476606905460357666015625;0.80337930974186411159365661660558544099330902099609375;-0.9190533864873196012723610692773945629596710205078125;-0.332463953329804773328959299760754220187664031982421875;0.462279811487102676448301963318954221904277801513671875;-0.96756671526222504109426836294005624949932098388671875;-0.200885959732653496256915559570188634097576141357421875;-0.01423059263944759407494178304887100239284336566925048828125;1.40293912576878643250211098347790539264678955078125;-0.83026811109425524559668474466889165341854095458984375;0.1702472352798871380041845213781925849616527557373046875;-0.70931219735333461695603318730718456208705902099609375;-1.26433865986847582263408185099251568317413330078125;-0.323365031628316035305914510900038294494152069091796875]
      mask Display: e = 0.06;c1 = [120 150 230]/255;c2 = ([120 150 230]+0)/383;c3 = ([120 150 230]+128)/383;patch([0 1 1 0],[0 0 1 1],c1);patch([0 1 1 1-e 1-e 0+e],[0 0 1 1-e 0+e 0+e],c2);patch([0 0 1 1-e 0+e 0+e],[0 1 1 1-e 1-e 0+e],c3);plot([0 1 1 0 0],[0 0 1 1 0]);disp('weights');
  "IW{5,3}(6,:)'" : Constant  Value=[-0.79428319918513945463445224959286861121654510498046875;-1.0427804228512524975513997560483403503894805908203125;0.486411744181387384333703494121436960995197296142578125;-0.44068666166099645931097938955645076930522918701171875;0.08498751778824940872336668462594388984143733978271484375;-0.54043989149282667394658119519590400159358978271484375;-0.75774013714248511508486672028084285557270050048828125;0.6347307195784941402649792507872916758060455322265625;0.413693669669123631482676728410297073423862457275390625;-1.1500351979482055231329695743625052273273468017578125;0.54801577353495056765808612908585928380489349365234375;-0.7424747261209974080742313162772916257381439208984375;-0.992785366273836178407918851007707417011260986328125;0.33912116910438483419198973933816887438297271728515625;0.291851394992376500514552617460140027105808258056640625;0.18261002637680479043780223946669138967990875244140625;0.08117182757240797019715472515599685721099376678466796875;0.062883074883410883249013068052590824663639068603515625;0.81893189205002137054378863467718474566936492919921875;0.791776856949927054785121072200126945972442626953125]
      mask Display: e = 0.06;c1 = [120 150 230]/255;c2 = ([120 150 230]+0)/383;c3 = ([120 150 230]+128)/383;patch([0 1 1 0],[0 0 1 1],c1);patch([0 1 1 1-e 1-e 0+e],[0 0 1 1-e 0+e 0+e],c2);patch([0 0 1 1-e 0+e 0+e],[0 1 1 1-e 1-e 0+e],c3);plot([0 1 1 0 0],[0 0 1 1 0]);disp('weights');
  "IW{5,3}(7,:)'" : Constant  Value=[-1.12422787591299933041000258526764810085296630859375;-0.2097785026464414059876872897802968509495258331298828125;0.491082305584683076471463891721214167773723602294921875;0.34493260635741374020568628111504949629306793212890625;0.70173383047816806357133145866100676357746124267578125;-0.84947547516357524433061598756466992199420928955078125;-1.5785390957905029996055645824526436626911163330078125;0.2338868169809479036214128200299455784261226654052734375;-0.2345684288954124341319840141295571811497211456298828125;0.53742220871835855167120143960346467792987823486328125;-0.404475432985955729581206696821027435362339019775390625;-0.51012726864364144052643723625806160271167755126953125;0.3684604322615658844597419374622404575347900390625;-0.87759650637207509138448813246213831007480621337890625;0.31749220961969271126434932739357464015483856201171875;0.98764552670645022747208940927521325647830963134765625;1.0398533730132368813059429157874546945095062255859375;1.502524150814558812072618820820935070514678955078125;0.269305693517003119641373132253647781908512115478515625;0.5626754059293637144634203650639392435550689697265625]
      mask Display: e = 0.06;c1 = [120 150 230]/255;c2 = ([120 150 230]+0)/383;c3 = ([120 150 230]+128)/383;patch([0 1 1 0],[0 0 1 1],c1);patch([0 1 1 1-e 1-e 0+e],[0 0 1 1-e 0+e 0+e],c2);patch([0 0 1 1-e 0+e 0+e],[0 1 1 1-e 1-e 0+e],c3);plot([0 1 1 0 0],[0 0 1 1 0]);disp('weights');
  "IW{5,3}(8,:)'" : Constant  Value=[0.238607229561909772730388112904620356857776641845703125;-0.786842679768771535719906751182861626148223876953125;0.12624363876869038048056381740025244653224945068359375;0.98963165975229916426769705140031874179840087890625;-0.7736601478587774582962310887523926794528961181640625;-0.61960214699662718995654131504124961793422698974609375;-0.4428287782758444368624850540072657167911529541015625;0.59754932179196840191792716723284684121608734130859375;0.469101952637317742844658141621039249002933502197265625;0.813468177418668947353808107436634600162506103515625;0.196836787283457714803347471388406120240688323974609375;1.0444060607363689907600701189949177205562591552734375;-1.1797245205586308625100855351774953305721282958984375;0.81325964419067753308212331830873154103755950927734375;-0.78978131450770827637342108573648147284984588623046875;-0.2319807373836731134719713054437306709587574005126953125;0.86564366816979154695133047425770200788974761962890625;0.50764602905011113609390349665773101150989532470703125;1.081100418578651467527151908143423497676849365234375;-0.70540533610873790149042861230554990470409393310546875]
      mask Display: e = 0.06;c1 = [120 150 230]/255;c2 = ([120 150 230]+0)/383;c3 = ([120 150 230]+128)/383;patch([0 1 1 0],[0 0 1 1],c1);patch([0 1 1 1-e 1-e 0+e],[0 0 1 1-e 0+e 0+e],c2);patch([0 0 1 1-e 0+e 0+e],[0 1 1 1-e 1-e 0+e],c3);plot([0 1 1 0 0],[0 0 1 1 0]);disp('weights');
  "IW{5,3}(9,:)'" : Constant  Value=[1.0370768809745147809309173680958338081836700439453125;-1.2034016323260614544921054402948357164859771728515625;-0.67956474126307331307117465257761068642139434814453125;1.03532584402798111256061019957996904850006103515625;-0.401180115225610478546514059416949748992919921875;-0.87672403252183428445931667738477699458599090576171875;0.5269404844504759211076816427521407604217529296875;0.38316922590776358870101603315561078488826751708984375;-0.58391135168300978275368606773554347455501556396484375;1.1899531865409864739291379009955562651157379150390625;-0.98113382916573621539413352365954779088497161865234375;-0.28879792358038314237234089887351728975772857666015625;0.204631046997458321268226200118078850209712982177734375;1.243809148881617421267264944617636501789093017578125;-1.0194625944999577971117332708672620356082916259765625;1.2302430754318514072309653784031979739665985107421875;0.7636855949973140322839526561438106000423431396484375;-0.4774900499118552854582731015398167073726654052734375;-1.1099524304615491221426282208994962275028228759765625;-0.437370101003972722164547803913592360913753509521484375]
      mask Display: e = 0.06;c1 = [120 150 230]/255;c2 = ([120 150 230]+0)/383;c3 = ([120 150 230]+128)/383;patch([0 1 1 0],[0 0 1 1],c1);patch([0 1 1 1-e 1-e 0+e],[0 0 1 1-e 0+e 0+e],c2);patch([0 0 1 1-e 0+e 0+e],[0 1 1 1-e 1-e 0+e],c3);plot([0 1 1 0 0],[0 0 1 1 0]);disp('weights');
  Mux : Mux  Inputs=10
      mask Display: e = 0.06;c1 = [120 150 230]/255;c2 = ([120 150 230]+0)/383;c3 = ([120 150 230]+128)/383;patch([0 1 1 0],[0 0 1 1],c1);patch([0 1 1 1-e 1-e 0+e],[0 0 1 1-e 0+e 0+e],c2);patch([0 0 1 1-e 0+e 0+e],[0 1 1 1-e 1-e 0+e],c3);plot([0 1 1 0 0],[0 0 1 1 0]);disp('Mux');
  dotprod{1..10} (10 alike) : neural/Weight Functions/dotprod
  "lz{5,3}" : Outport
      mask Display: e = 0.06;c1 = [120 230 180]/255;c2 = ([120 230 180]+0)/(256+128);c3 = ([120 230 180]+128)/(256+128);patch([0 1 1 0],[0 0 1 1],c1);patch([0 1 1 1-e 1-e 0+e],[0 0 1 1-e 0+e 0+e],c2);patch([0 0 1 1-e 0+e 0+e],[0 1 1 1-e 1-e 0+e],c3);plot([0 1 1 0 0],[0 0 1 1 0]);
  wires:
  "IW{5,3}(1,:)'"/1 -> dotprod1/1
  "ad{5,3}"/1 -> dotprod1/2, dotprod2/2, dotprod3/2, dotprod4/2, dotprod5/2, dotprod6/2, dotprod7/2, dotprod8/2, dotprod9/2, dotprod10/2
  dotprod1/1 -> Mux/1
  "IW{5,3}(2,:)'"/1 -> dotprod2/1
  dotprod2/1 -> Mux/2
  "IW{5,3}(3,:)'"/1 -> dotprod3/1
  dotprod3/1 -> Mux/3
  "IW{5,3}(4,:)'"/1 -> dotprod4/1
  dotprod4/1 -> Mux/4
  "IW{5,3}(5,:)'"/1 -> dotprod5/1
  dotprod5/1 -> Mux/5
  "IW{5,3}(6,:)'"/1 -> dotprod6/1
  dotprod6/1 -> Mux/6
  "IW{5,3}(7,:)'"/1 -> dotprod7/1
  dotprod7/1 -> Mux/7
  "IW{5,3}(8,:)'"/1 -> dotprod8/1
  dotprod8/1 -> Mux/8
  "IW{5,3}(9,:)'"/1 -> dotprod9/1
  dotprod9/1 -> Mux/9
  "IW{5,3}(10,:)'"/1 -> dotprod10/1
  dotprod10/1 -> Mux/10
  Mux/1 -> "lz{5,3}"/1
